simulink model "Framework"  (R2017b)
settings: Solver=ode1  StartTime=0.0  StopTime=Inf  FixedStep=0.001  RelTol=1e-3
PostLoadFcn:
  | , if any(exist('dsrtsu_mdlpostloadfcn', 'file') == [2, 3, 6]), try dsrtsu_mdlpostloadfcn('Execute', bdroot); catch fprintf('Error in PostLoadFcn (dsrtsu_mdlpostloadfcn) for model "%s":\n %s\n', bdroot, lasterr); end, end,
InitFcn:
  | Parameter_INIT
undefined symbols (not defined in the file or in its folder): drive, motor
libraries: rtican x46, simulink x8, neural x1
(part 9 of 10)

== system Framework/rpm FL ==
  Front_Motor_Enable : Inport
  Motor_Output_FL : Inport  Port=2
  Gain1 : Gain
  Terminator_2 : Terminator
  Terminator_3 : Terminator
  Terminator_4 : Terminator
  Transmit OK Detection1 : Subsystem
  _CAN_TYPE1_TX_M1_C2 : rtican/RTICAN Transmit (TX)   Reserved1=[]  Reserved2=[]  Reserved3=[]  Reserved4=[]  SfcnMessage=[]  Msg_Struct=[]  BoardTypeNo=[]  BoardNo=[]  ChannelNo=[]  Parameters=[]  DialogFcn=[]  UnitName=[]  Revision=[]  UnitValues=[]  DSProperties=struct('RTI',struct('Version',uint32(5),'BlockType',struct('isSLSource',uint8(1),'isSLSink',uint8(1),'isHWSource',uint8(0),'isHWSink',uint8(0),'isSetup',uint8(0),'isInline',uint8(1),'isNonInline',uint8(0),'isInterrupt',uint8(0),'isChannelwise',uint8(0)),'IOBoardType','RTICAN','UnitType','MESSAGE','Identifier','TX','DialogType','MSVC','BlockSet','RTICAN','SlaveProcessor','CAN'))  RTIBlockInterface=struct('InputPortsWidth',int32(1),'InputPortsActive',1,'InputPortsName',{{'RPM'}},'InputPortsDataType',{{'SS_DOUBLE'}},'OutputPortsWidth',int32([1 1 1 1]),'OutputPortsActive',[1 1 1 1],'OutputPortsName',{{['TX status'],['TX time'],['TX delta time'],['TX delay time']}},'DialogFcn','rtican_message_interface_gui','BlockDisplay',{{'','center'}},'IconTransparency','on','InitLevel',3,'BlockName',struct('Token',{{'CAN_TYPE','_TX_M','_C'}},'BlockParam',{{'BoardTypeNo','BoardNo','ChannelNo'}}),'SampleTime',{{-1}},'TriggerPort',{{'none'}},'EnablePort',{{'yes'}})  RTIBlockParameters=struct('BoardTypeNo',{{1,'OFF',[]}},'BoardNo',{{1,'ON',[1 16]}},'ChannelNo',{{2,'ON',[1 2]}},'Parameters',{{struct('DataFileSupport',struct('DataFileSelectedMaster',0,'DataFileSelectedLocal',0,'DataFileName',['<no datafile support>|'],'DataFileDate','','SelectedFile',['<no file selected>']),'Options',struct('StatusSelected',1,'TimeSelected',1,'DeltaTimeSelected',1,'DelayTimeSelected',1,'DelayTimeTXCommandSelected',0,'EncodeSetUnusedBitsToOne',0,'EnableMsgLoopback',0,'TriggerPort',struct('Selected',0,'TriggerType',0),'EnablePortSelected',1,'SignalOnPortnameSelected',1,'UserCoding',struct('Selected',0,'InterfaceFile','UserEncodingFile','FcnName','UserEncodeFcn','InportSelected',0,'InportWidth',1,'OutportSelected',0,'OutportWidth',1),'TerminationMsg',struct('Selected',0,'Byte0_7','0'),'InitialMsg',struct('Selected',0,'Byte0_7','0')),'Message',struct('MsgOnBlocknameSelected',0,'MsgName',['TX Message'],'MsgIdFormat',1,'MsgId',780,'MsgLength',4,'NumSignals',1,'SampleTime',-1,'StartTime',struct('Selected',0,'Value',2),'AutoRepeatTime',struct('Selected',0,'Value',0.1),'Timeout',struct('Selected',0,'Value',0.1),'DelayTime',struct('Selected',0,'Value',0.1),'Signal',struct('SgnName','RPM','SgnStartBit',0,'SgnLength',32,'SgnType',0,'ModeValue',-1,'DataType',1,'ByteLayout',1,'Factor',1,'Offset',0,'SgnComment',{{''}},'SgnUnit','','Min',0,'Max',255,'SLDataType','SS_DOUBLE'),'MsgIdNumFormat',1,'MsgComment',{{''}}),'Version',1.2,'general',struct('isFromLib',0)),'OFF',[]}},'GroupId',{{struct('Group',{{'RTICAN'}},'No',2,'Behavior',{{'NAMECHANGE'}},'BlockType',{{'SINK'}},'NameChangeFlag',0),'OFF',[]}},'SFcnRTICANMessage',{{struct('MsgType','TX','SFcnPortType','Scalar','MsgName',['TX Message'],'MsgIdFormat','XTD','MsgId',780,'MsgLength',4,'NumSignals',1,'SampleTime',-1,'StartTime',struct('Selected','no','Value',2),'AutoRepeatTime',struct('Selected','no','Value',0.1),'Timeout',struct('Selected','no','Value',0.1),'Signal',struct('SgnName','RPM','SgnStartBit',0,'SgnLength',32,'SgnType','standard','ModeValue',-1,'DataType',['signed int'],'ByteLayout',['big endian'],'Factor',1,'Offset',0,'SLDataType','SS_DOUBLE'),'StatusSelected','yes','TimeSelected','yes','DeltaTimeSelected','yes','DelayTimeSelected','yes','DelayTimeTXCommandSelected','no','EncodeSetUnusedBitsToOne','no','EnableMsgLoopback','no','TriggerPort',struct('Selected','no','TriggerType',0),'EnablePortSelected','yes','UserCoding',struct('Selected','no','InterfaceFile','UserEncodingFile','FcnName','UserEncodeFcn','InportSelected','no','InportWidth',1,'OutportSelected','no','OutportWidth',1),'TerminationMsg',struct('Selected','no','Byte0','0x00','Byte1','0x00','Byte2','0x00','Byte3','0x00','Byte4','0x00','Byte5','0x00','Byte6','0x00','Byte7','0x00'),'InitialMsg',struct('Selected','no','Byte0','0x00','Byte1','0x00','Byte2','0x00','Byte3','0x00','Byte4','0x00','Byte5','0x00','Byte6','0x00','Byte7','0x00'),'BoardType','DS1','BoardNo',1,'ControllerNo',2),'OFF',[]}},'TLCFileName',{{'rtican_tx_message','OFF',[]}})  RTISFcnParameters=struct('SFcnRTICANMessage','struct','TLCFileName','char')  RTIBlockParaDefault=struct('BoardTypeNo',4302,'BoardNo',1,'ChannelNo',1,'Parameters',struct('DataFileSupport',struct('DataFileSelectedMaster',0,'DataFileSelectedLocal',0,'DataFileName','','DataFileDate','','SelectedFile',['<no file selected>']),'Options',struct('StatusSelected',1,'TimeSelected',1,'DeltaTimeSelected',1,'DelayTimeSelected',1,'DelayTimeTXCommandSelected',0,'EncodeSetUnusedBitsToOne',0,'EnableMsgLoopback',0,'TriggerPort',struct('Selected',0,'TriggerType','rising'),'EnablePortSelected',0,'SignalOnPortnameSelected',1,'UserCoding',struct('Selected',0,'InterfaceFile','UserEncodingFile','FcnName','UserEncodeFcn','InportSelected',0,'InportWidth',1,'OutportSelected',0,'OutportWidth',1),'TerminationMsg',struct('Selected',0,'Byte0_7','0'),'InitialMsg',struct('Selected',0,'Byte0_7','0')),'Message',struct('MsgOnBlocknameSelected',0,'MsgName',['TX Message'],'MsgIdFormat',0,'MsgId',100,'MsgLength',8,'NumSignals',1,'SampleTime',-1,'StartTime',struct('Selected',0,'Value',0),'AutoRepeatTime',struct('Selected',0,'Value',0.1),'Timeout',struct('Selected',0,'Value',0.1),'DelayTime',struct('Selected',0,'Value',0.1),'Signal',struct('SgnName',['TX signal'],'SgnStartBit',0,'SgnLength',8,'SgnType',0,'ModeValue',-1,'DataType',0,'SLDataType','SS_DOUBLE','ByteLayout',0,'Factor',1,'Offset',0,'Min',0,'Max',255,'SgnComment',{{}},'SgnUnit',''),'MsgIdNumFormat',0,'MsgComment',{{''}}),'Version',1.2,'general',struct('isFromLib',1)),'GroupId',struct('Group',{{'RTICAN'}},'No',1,'Behavior',{{'NAMECHANGE'}},'BlockType',{{'SINK'}},'NameChangeFlag',0),'SFcnRTICANMessage',struct('MsgType','TX','MsgName',['TX Message'],'MsgIdFormat','STD','MsgId',100,'MsgLength',2,'NumSignals',1,'SampleTime',-1,'StartTime',struct('Selected','no','Value',0),'AutoRepeatTime',struct('Selected','no','Value',0.1),'Timeout',struct('Selected','no','Value',0.1),'DelayTime',struct('Selected','no','Value',0.1),'Signal',struct('SgnName',['TX signal'],'SgnStartBit',0,'SgnLength',8,'SgnType','standard','ModeValue',-1,'DataType',['unsigned int'],'ByteLayout',['little endian'],'SLDataType','SS_DOUBLE','Factor',1,'Offset',0),'StatusSelected','yes','TimeSelected','yes','DeltaTimeSelected','yes','DelayTimeSelected','yes','EnablePortSelected','no','EnableMsgLoopback','no','DelayTimeTXCommandSelected','no','EncodeSetUnusedBitsToOne','no','UserCoding',struct('Selected','no','InterfaceFile','UserDecodingFile','FcnName','UserDecodeFcn','InportSelected','no','InportWidth',1,'OutportSelected','no','OutportWidth',1),'TerminationMsg',struct('Selected','no','Byte0','0x00','Byte1','0x00','Byte2','0x00','Byte3','0x00','Byte4','0x00','Byte5','0x00','Byte6','0x00','Byte7','0x00'),'InitialMsg',struct('Selected','no','Byte0','0x00','Byte1','0x00','Byte2','0x00','Byte3','0x00','Byte4','0x00','Byte5','0x00','Byte6','0x00','Byte7','0x00'),'TriggerPort',struct('Selected','no','TriggerType','rising'),'BoardType','DS4302','BoardNo',1,'ControllerNo',1,'SFcnPortType','Scalar'),'TLCFileName','rtican_tx_message')
      settings: AttributesFormatString=Group Id: RTICAN2\n  SourceProductName=dSPACE RTI CAN Blockset
  wires:
  Front_Motor_Enable/1 -> _CAN_TYPE1_TX_M1_C2/Enable  "Front_Motor_Enable"
  Motor_Output_FL/1 -> Gain1/1  "Motor_Output_FR"
  _CAN_TYPE1_TX_M1_C2/4 -> Terminator_3/1
  _CAN_TYPE1_TX_M1_C2/3 -> Transmit OK Detection1/2(TX delta time)
  _CAN_TYPE1_TX_M1_C2/1 -> Transmit OK Detection1/1(TX status)
  _CAN_TYPE1_TX_M1_C2/2 -> Terminator_2/1
  Transmit OK Detection1/1(TX Warn) -> Terminator_4/1
  Gain1/1 -> _CAN_TYPE1_TX_M1_C2/1

== system Framework/rpm FR ==
  Front_Motor_Enable : Inport
  Motor_Output_FR : Inport  Port=2
  Gain1 : Gain
  Terminator_2 : Terminator
  Terminator_3 : Terminator
  Terminator_4 : Terminator
  Transmit OK Detection1 : Subsystem
  _CAN_TYPE1_TX_M1_C2 : rtican/RTICAN Transmit (TX)   Reserved1=[]  Reserved2=[]  Reserved3=[]  Reserved4=[]  SfcnMessage=[]  Msg_Struct=[]  BoardTypeNo=[]  BoardNo=[]  ChannelNo=[]  Parameters=[]  DialogFcn=[]  UnitName=[]  Revision=[]  UnitValues=[]  DSProperties=struct('RTI',struct('Version',uint32(5),'BlockType',struct('isSLSource',uint8(1),'isSLSink',uint8(1),'isHWSource',uint8(0),'isHWSink',uint8(0),'isSetup',uint8(0),'isInline',uint8(1),'isNonInline',uint8(0),'isInterrupt',uint8(0),'isChannelwise',uint8(0)),'IOBoardType','RTICAN','UnitType','MESSAGE','Identifier','TX','DialogType','MSVC','BlockSet','RTICAN','SlaveProcessor','CAN'))  RTIBlockInterface=struct('InputPortsWidth',int32(1),'InputPortsActive',1,'InputPortsName',{{'RPM'}},'InputPortsDataType',{{'SS_DOUBLE'}},'OutputPortsWidth',int32([1 1 1 1]),'OutputPortsActive',[1 1 1 1],'OutputPortsName',{{['TX status'],['TX time'],['TX delta time'],['TX delay time']}},'DialogFcn','rtican_message_interface_gui','BlockDisplay',{{'','center'}},'IconTransparency','on','InitLevel',3,'BlockName',struct('Token',{{'CAN_TYPE','_TX_M','_C'}},'BlockParam',{{'BoardTypeNo','BoardNo','ChannelNo'}}),'SampleTime',{{-1}},'TriggerPort',{{'none'}},'EnablePort',{{'yes'}})  RTIBlockParameters=struct('BoardTypeNo',{{1,'OFF',[]}},'BoardNo',{{1,'ON',[1 16]}},'ChannelNo',{{2,'ON',[1 2]}},'Parameters',{{struct('DataFileSupport',struct('DataFileSelectedMaster',0,'DataFileSelectedLocal',0,'DataFileName',['<no datafile support>|'],'DataFileDate','','SelectedFile',['<no file selected>']),'Options',struct('StatusSelected',1,'TimeSelected',1,'DeltaTimeSelected',1,'DelayTimeSelected',1,'DelayTimeTXCommandSelected',0,'EncodeSetUnusedBitsToOne',0,'EnableMsgLoopback',0,'TriggerPort',struct('Selected',0,'TriggerType',0),'EnablePortSelected',1,'SignalOnPortnameSelected',1,'UserCoding',struct('Selected',0,'InterfaceFile','UserEncodingFile','FcnName','UserEncodeFcn','InportSelected',0,'InportWidth',1,'OutportSelected',0,'OutportWidth',1),'TerminationMsg',struct('Selected',0,'Byte0_7','0'),'InitialMsg',struct('Selected',0,'Byte0_7','0')),'Message',struct('MsgOnBlocknameSelected',0,'MsgName',['TX Message'],'MsgIdFormat',1,'MsgId',795,'MsgLength',4,'NumSignals',1,'SampleTime',-1,'StartTime',struct('Selected',0,'Value',2),'AutoRepeatTime',struct('Selected',0,'Value',0.1),'Timeout',struct('Selected',0,'Value',0.1),'DelayTime',struct('Selected',0,'Value',0.1),'Signal',struct('SgnName','RPM','SgnStartBit',0,'SgnLength',32,'SgnType',0,'ModeValue',-1,'DataType',1,'ByteLayout',1,'Factor',1,'Offset',0,'SgnComment',{{''}},'SgnUnit','','Min',0,'Max',255,'SLDataType','SS_DOUBLE'),'MsgIdNumFormat',1,'MsgComment',{{''}}),'Version',1.2,'general',struct('isFromLib',0)),'OFF',[]}},'GroupId',{{struct('Group',{{'RTICAN'}},'No',2,'Behavior',{{'NAMECHANGE'}},'BlockType',{{'SINK'}},'NameChangeFlag',0),'OFF',[]}},'SFcnRTICANMessage',{{struct('MsgType','TX','SFcnPortType','Scalar','MsgName',['TX Message'],'MsgIdFormat','XTD','MsgId',795,'MsgLength',4,'NumSignals',1,'SampleTime',-1,'StartTime',struct('Selected','no','Value',2),'AutoRepeatTime',struct('Selected','no','Value',0.1),'Timeout',struct('Selected','no','Value',0.1),'Signal',struct('SgnName','RPM','SgnStartBit',0,'SgnLength',32,'SgnType','standard','ModeValue',-1,'DataType',['signed int'],'ByteLayout',['big endian'],'Factor',1,'Offset',0,'SLDataType','SS_DOUBLE'),'StatusSelected','yes','TimeSelected','yes','DeltaTimeSelected','yes','DelayTimeSelected','yes','DelayTimeTXCommandSelected','no','EncodeSetUnusedBitsToOne','no','EnableMsgLoopback','no','TriggerPort',struct('Selected','no','TriggerType',0),'EnablePortSelected','yes','UserCoding',struct('Selected','no','InterfaceFile','UserEncodingFile','FcnName','UserEncodeFcn','InportSelected','no','InportWidth',1,'OutportSelected','no','OutportWidth',1),'TerminationMsg',struct('Selected','no','Byte0','0x00','Byte1','0x00','Byte2','0x00','Byte3','0x00','Byte4','0x00','Byte5','0x00','Byte6','0x00','Byte7','0x00'),'InitialMsg',struct('Selected','no','Byte0','0x00','Byte1','0x00','Byte2','0x00','Byte3','0x00','Byte4','0x00','Byte5','0x00','Byte6','0x00','Byte7','0x00'),'BoardType','DS1','BoardNo',1,'ControllerNo',2),'OFF',[]}},'TLCFileName',{{'rtican_tx_message','OFF',[]}})  RTISFcnParameters=struct('SFcnRTICANMessage','struct','TLCFileName','char')  RTIBlockParaDefault=struct('BoardTypeNo',4302,'BoardNo',1,'ChannelNo',1,'Parameters',struct('DataFileSupport',struct('DataFileSelectedMaster',0,'DataFileSelectedLocal',0,'DataFileName','','DataFileDate','','SelectedFile',['<no file selected>']),'Options',struct('StatusSelected',1,'TimeSelected',1,'DeltaTimeSelected',1,'DelayTimeSelected',1,'DelayTimeTXCommandSelected',0,'EncodeSetUnusedBitsToOne',0,'EnableMsgLoopback',0,'TriggerPort',struct('Selected',0,'TriggerType','rising'),'EnablePortSelected',0,'SignalOnPortnameSelected',1,'UserCoding',struct('Selected',0,'InterfaceFile','UserEncodingFile','FcnName','UserEncodeFcn','InportSelected',0,'InportWidth',1,'OutportSelected',0,'OutportWidth',1),'TerminationMsg',struct('Selected',0,'Byte0_7','0'),'InitialMsg',struct('Selected',0,'Byte0_7','0')),'Message',struct('MsgOnBlocknameSelected',0,'MsgName',['TX Message'],'MsgIdFormat',0,'MsgId',100,'MsgLength',8,'NumSignals',1,'SampleTime',-1,'StartTime',struct('Selected',0,'Value',0),'AutoRepeatTime',struct('Selected',0,'Value',0.1),'Timeout',struct('Selected',0,'Value',0.1),'DelayTime',struct('Selected',0,'Value',0.1),'Signal',struct('SgnName',['TX signal'],'SgnStartBit',0,'SgnLength',8,'SgnType',0,'ModeValue',-1,'DataType',0,'SLDataType','SS_DOUBLE','ByteLayout',0,'Factor',1,'Offset',0,'Min',0,'Max',255,'SgnComment',{{}},'SgnUnit',''),'MsgIdNumFormat',0,'MsgComment',{{''}}),'Version',1.2,'general',struct('isFromLib',1)),'GroupId',struct('Group',{{'RTICAN'}},'No',1,'Behavior',{{'NAMECHANGE'}},'BlockType',{{'SINK'}},'NameChangeFlag',0),'SFcnRTICANMessage',struct('MsgType','TX','MsgName',['TX Message'],'MsgIdFormat','STD','MsgId',100,'MsgLength',2,'NumSignals',1,'SampleTime',-1,'StartTime',struct('Selected','no','Value',0),'AutoRepeatTime',struct('Selected','no','Value',0.1),'Timeout',struct('Selected','no','Value',0.1),'DelayTime',struct('Selected','no','Value',0.1),'Signal',struct('SgnName',['TX signal'],'SgnStartBit',0,'SgnLength',8,'SgnType','standard','ModeValue',-1,'DataType',['unsigned int'],'ByteLayout',['little endian'],'SLDataType','SS_DOUBLE','Factor',1,'Offset',0),'StatusSelected','yes','TimeSelected','yes','DeltaTimeSelected','yes','DelayTimeSelected','yes','EnablePortSelected','no','EnableMsgLoopback','no','DelayTimeTXCommandSelected','no','EncodeSetUnusedBitsToOne','no','UserCoding',struct('Selected','no','InterfaceFile','UserDecodingFile','FcnName','UserDecodeFcn','InportSelected','no','InportWidth',1,'OutportSelected','no','OutportWidth',1),'TerminationMsg',struct('Selected','no','Byte0','0x00','Byte1','0x00','Byte2','0x00','Byte3','0x00','Byte4','0x00','Byte5','0x00','Byte6','0x00','Byte7','0x00'),'InitialMsg',struct('Selected','no','Byte0','0x00','Byte1','0x00','Byte2','0x00','Byte3','0x00','Byte4','0x00','Byte5','0x00','Byte6','0x00','Byte7','0x00'),'TriggerPort',struct('Selected','no','TriggerType','rising'),'BoardType','DS4302','BoardNo',1,'ControllerNo',1,'SFcnPortType','Scalar'),'TLCFileName','rtican_tx_message')
      settings: AttributesFormatString=Group Id: RTICAN2\n  SourceProductName=dSPACE RTI CAN Blockset
  wires:
  Front_Motor_Enable/1 -> _CAN_TYPE1_TX_M1_C2/Enable  "Front_Motor_Enable"
  Motor_Output_FR/1 -> Gain1/1  "Motor_Output_FR"
  _CAN_TYPE1_TX_M1_C2/4 -> Terminator_3/1
  _CAN_TYPE1_TX_M1_C2/3 -> Transmit OK Detection1/2(TX delta time)
  _CAN_TYPE1_TX_M1_C2/1 -> Transmit OK Detection1/1(TX status)
  _CAN_TYPE1_TX_M1_C2/2 -> Terminator_2/1
  Transmit OK Detection1/1(TX Warn) -> Terminator_4/1
  Gain1/1 -> _CAN_TYPE1_TX_M1_C2/1

== system Framework/rpm RL ==
  Front_Motor_Enable : Inport
  Motor_Output_RL : Inport  Port=2
  Gain1 : Gain
  Terminator_2 : Terminator
  Terminator_3 : Terminator
  Terminator_4 : Terminator
  Transmit OK Detection1 : Subsystem
  _CAN_TYPE1_TX_M1_C2 : rtican/RTICAN Transmit (TX)   Reserved1=[]  Reserved2=[]  Reserved3=[]  Reserved4=[]  SfcnMessage=[]  Msg_Struct=[]  BoardTypeNo=[]  BoardNo=[]  ChannelNo=[]  Parameters=[]  DialogFcn=[]  UnitName=[]  Revision=[]  UnitValues=[]  DSProperties=struct('RTI',struct('Version',uint32(5),'BlockType',struct('isSLSource',uint8(1),'isSLSink',uint8(1),'isHWSource',uint8(0),'isHWSink',uint8(0),'isSetup',uint8(0),'isInline',uint8(1),'isNonInline',uint8(0),'isInterrupt',uint8(0),'isChannelwise',uint8(0)),'IOBoardType','RTICAN','UnitType','MESSAGE','Identifier','TX','DialogType','MSVC','BlockSet','RTICAN','SlaveProcessor','CAN'))  RTIBlockInterface=struct('InputPortsWidth',int32(1),'InputPortsActive',1,'InputPortsName',{{'RPM'}},'InputPortsDataType',{{'SS_DOUBLE'}},'OutputPortsWidth',int32([1 1 1 1]),'OutputPortsActive',[1 1 1 1],'OutputPortsName',{{['TX status'],['TX time'],['TX delta time'],['TX delay time']}},'DialogFcn','rtican_message_interface_gui','BlockDisplay',{{'','center'}},'IconTransparency','on','InitLevel',3,'BlockName',struct('Token',{{'CAN_TYPE','_TX_M','_C'}},'BlockParam',{{'BoardTypeNo','BoardNo','ChannelNo'}}),'SampleTime',{{-1}},'TriggerPort',{{'none'}},'EnablePort',{{'yes'}})  RTIBlockParameters=struct('BoardTypeNo',{{1,'OFF',[]}},'BoardNo',{{1,'ON',[1 16]}},'ChannelNo',{{2,'ON',[1 2]}},'Parameters',{{struct('DataFileSupport',struct('DataFileSelectedMaster',0,'DataFileSelectedLocal',0,'DataFileName',['<no datafile support>|'],'DataFileDate','','SelectedFile',['<no file selected>']),'Options',struct('StatusSelected',1,'TimeSelected',1,'DeltaTimeSelected',1,'DelayTimeSelected',1,'DelayTimeTXCommandSelected',0,'EncodeSetUnusedBitsToOne',0,'EnableMsgLoopback',0,'TriggerPort',struct('Selected',0,'TriggerType',0),'EnablePortSelected',1,'SignalOnPortnameSelected',1,'UserCoding',struct('Selected',0,'InterfaceFile','UserEncodingFile','FcnName','UserEncodeFcn','InportSelected',0,'InportWidth',1,'OutportSelected',0,'OutportWidth',1),'TerminationMsg',struct('Selected',0,'Byte0_7','0'),'InitialMsg',struct('Selected',0,'Byte0_7','0')),'Message',struct('MsgOnBlocknameSelected',0,'MsgName',['TX Message'],'MsgIdFormat',1,'MsgId',848,'MsgLength',4,'NumSignals',1,'SampleTime',-1,'StartTime',struct('Selected',0,'Value',2),'AutoRepeatTime',struct('Selected',0,'Value',0.1),'Timeout',struct('Selected',0,'Value',0.1),'DelayTime',struct('Selected',0,'Value',0.1),'Signal',struct('SgnName','RPM','SgnStartBit',0,'SgnLength',32,'SgnType',0,'ModeValue',-1,'DataType',1,'ByteLayout',1,'Factor',1,'Offset',0,'SgnComment',{{''}},'SgnUnit','','Min',0,'Max',255,'SLDataType','SS_DOUBLE'),'MsgIdNumFormat',1,'MsgComment',{{''}}),'Version',1.2,'general',struct('isFromLib',0)),'OFF',[]}},'GroupId',{{struct('Group',{{'RTICAN'}},'No',2,'Behavior',{{'NAMECHANGE'}},'BlockType',{{'SINK'}},'NameChangeFlag',0),'OFF',[]}},'SFcnRTICANMessage',{{struct('MsgType','TX','SFcnPortType','Scalar','MsgName',['TX Message'],'MsgIdFormat','XTD','MsgId',848,'MsgLength',4,'NumSignals',1,'SampleTime',-1,'StartTime',struct('Selected','no','Value',2),'AutoRepeatTime',struct('Selected','no','Value',0.1),'Timeout',struct('Selected','no','Value',0.1),'Signal',struct('SgnName','RPM','SgnStartBit',0,'SgnLength',32,'SgnType','standard','ModeValue',-1,'DataType',['signed int'],'ByteLayout',['big endian'],'Factor',1,'Offset',0,'SLDataType','SS_DOUBLE'),'StatusSelected','yes','TimeSelected','yes','DeltaTimeSelected','yes','DelayTimeSelected','yes','DelayTimeTXCommandSelected','no','EncodeSetUnusedBitsToOne','no','EnableMsgLoopback','no','TriggerPort',struct('Selected','no','TriggerType',0),'EnablePortSelected','yes','UserCoding',struct('Selected','no','InterfaceFile','UserEncodingFile','FcnName','UserEncodeFcn','InportSelected','no','InportWidth',1,'OutportSelected','no','OutportWidth',1),'TerminationMsg',struct('Selected','no','Byte0','0x00','Byte1','0x00','Byte2','0x00','Byte3','0x00','Byte4','0x00','Byte5','0x00','Byte6','0x00','Byte7','0x00'),'InitialMsg',struct('Selected','no','Byte0','0x00','Byte1','0x00','Byte2','0x00','Byte3','0x00','Byte4','0x00','Byte5','0x00','Byte6','0x00','Byte7','0x00'),'BoardType','DS1','BoardNo',1,'ControllerNo',2),'OFF',[]}},'TLCFileName',{{'rtican_tx_message','OFF',[]}})  RTISFcnParameters=struct('SFcnRTICANMessage','struct','TLCFileName','char')  RTIBlockParaDefault=struct('BoardTypeNo',4302,'BoardNo',1,'ChannelNo',1,'Parameters',struct('DataFileSupport',struct('DataFileSelectedMaster',0,'DataFileSelectedLocal',0,'DataFileName','','DataFileDate','','SelectedFile',['<no file selected>']),'Options',struct('StatusSelected',1,'TimeSelected',1,'DeltaTimeSelected',1,'DelayTimeSelected',1,'DelayTimeTXCommandSelected',0,'EncodeSetUnusedBitsToOne',0,'EnableMsgLoopback',0,'TriggerPort',struct('Selected',0,'TriggerType','rising'),'EnablePortSelected',0,'SignalOnPortnameSelected',1,'UserCoding',struct('Selected',0,'InterfaceFile','UserEncodingFile','FcnName','UserEncodeFcn','InportSelected',0,'InportWidth',1,'OutportSelected',0,'OutportWidth',1),'TerminationMsg',struct('Selected',0,'Byte0_7','0'),'InitialMsg',struct('Selected',0,'Byte0_7','0')),'Message',struct('MsgOnBlocknameSelected',0,'MsgName',['TX Message'],'MsgIdFormat',0,'MsgId',100,'MsgLength',8,'NumSignals',1,'SampleTime',-1,'StartTime',struct('Selected',0,'Value',0),'AutoRepeatTime',struct('Selected',0,'Value',0.1),'Timeout',struct('Selected',0,'Value',0.1),'DelayTime',struct('Selected',0,'Value',0.1),'Signal',struct('SgnName',['TX signal'],'SgnStartBit',0,'SgnLength',8,'SgnType',0,'ModeValue',-1,'DataType',0,'SLDataType','SS_DOUBLE','ByteLayout',0,'Factor',1,'Offset',0,'Min',0,'Max',255,'SgnComment',{{}},'SgnUnit',''),'MsgIdNumFormat',0,'MsgComment',{{''}}),'Version',1.2,'general',struct('isFromLib',1)),'GroupId',struct('Group',{{'RTICAN'}},'No',1,'Behavior',{{'NAMECHANGE'}},'BlockType',{{'SINK'}},'NameChangeFlag',0),'SFcnRTICANMessage',struct('MsgType','TX','MsgName',['TX Message'],'MsgIdFormat','STD','MsgId',100,'MsgLength',2,'NumSignals',1,'SampleTime',-1,'StartTime',struct('Selected','no','Value',0),'AutoRepeatTime',struct('Selected','no','Value',0.1),'Timeout',struct('Selected','no','Value',0.1),'DelayTime',struct('Selected','no','Value',0.1),'Signal',struct('SgnName',['TX signal'],'SgnStartBit',0,'SgnLength',8,'SgnType','standard','ModeValue',-1,'DataType',['unsigned int'],'ByteLayout',['little endian'],'SLDataType','SS_DOUBLE','Factor',1,'Offset',0),'StatusSelected','yes','TimeSelected','yes','DeltaTimeSelected','yes','DelayTimeSelected','yes','EnablePortSelected','no','EnableMsgLoopback','no','DelayTimeTXCommandSelected','no','EncodeSetUnusedBitsToOne','no','UserCoding',struct('Selected','no','InterfaceFile','UserDecodingFile','FcnName','UserDecodeFcn','InportSelected','no','InportWidth',1,'OutportSelected','no','OutportWidth',1),'TerminationMsg',struct('Selected','no','Byte0','0x00','Byte1','0x00','Byte2','0x00','Byte3','0x00','Byte4','0x00','Byte5','0x00','Byte6','0x00','Byte7','0x00'),'InitialMsg',struct('Selected','no','Byte0','0x00','Byte1','0x00','Byte2','0x00','Byte3','0x00','Byte4','0x00','Byte5','0x00','Byte6','0x00','Byte7','0x00'),'TriggerPort',struct('Selected','no','TriggerType','rising'),'BoardType','DS4302','BoardNo',1,'ControllerNo',1,'SFcnPortType','Scalar'),'TLCFileName','rtican_tx_message')
      settings: AttributesFormatString=Group Id: RTICAN2\n  SourceProductName=dSPACE RTI CAN Blockset
  wires:
  Front_Motor_Enable/1 -> _CAN_TYPE1_TX_M1_C2/Enable  "Front_Motor_Enable"
  Motor_Output_RL/1 -> Gain1/1  "Motor_Output_FR"
  _CAN_TYPE1_TX_M1_C2/4 -> Terminator_3/1
  _CAN_TYPE1_TX_M1_C2/3 -> Transmit OK Detection1/2(TX delta time)
  _CAN_TYPE1_TX_M1_C2/1 -> Transmit OK Detection1/1(TX status)
  _CAN_TYPE1_TX_M1_C2/2 -> Terminator_2/1
  Transmit OK Detection1/1(TX Warn) -> Terminator_4/1
  Gain1/1 -> _CAN_TYPE1_TX_M1_C2/1

== system Framework/rpm RR ==
  Front_Motor_Enable : Inport
  Motor_Output_RR : Inport  Port=2
  Gain1 : Gain
  Terminator_2 : Terminator
  Terminator_3 : Terminator
  Terminator_4 : Terminator
  Transmit OK Detection1 : Subsystem
  _CAN_TYPE1_TX_M1_C2 : rtican/RTICAN Transmit (TX)   Reserved1=[]  Reserved2=[]  Reserved3=[]  Reserved4=[]  SfcnMessage=[]  Msg_Struct=[]  BoardTypeNo=[]  BoardNo=[]  ChannelNo=[]  Parameters=[]  DialogFcn=[]  UnitName=[]  Revision=[]  UnitValues=[]  DSProperties=struct('RTI',struct('Version',uint32(5),'BlockType',struct('isSLSource',uint8(1),'isSLSink',uint8(1),'isHWSource',uint8(0),'isHWSink',uint8(0),'isSetup',uint8(0),'isInline',uint8(1),'isNonInline',uint8(0),'isInterrupt',uint8(0),'isChannelwise',uint8(0)),'IOBoardType','RTICAN','UnitType','MESSAGE','Identifier','TX','DialogType','MSVC','BlockSet','RTICAN','SlaveProcessor','CAN'))  RTIBlockInterface=struct('InputPortsWidth',int32(1),'InputPortsActive',1,'InputPortsName',{{'RPM'}},'InputPortsDataType',{{'SS_DOUBLE'}},'OutputPortsWidth',int32([1 1 1 1]),'OutputPortsActive',[1 1 1 1],'OutputPortsName',{{['TX status'],['TX time'],['TX delta time'],['TX delay time']}},'DialogFcn','rtican_message_interface_gui','BlockDisplay',{{'','center'}},'IconTransparency','on','InitLevel',3,'BlockName',struct('Token',{{'CAN_TYPE','_TX_M','_C'}},'BlockParam',{{'BoardTypeNo','BoardNo','ChannelNo'}}),'SampleTime',{{-1}},'TriggerPort',{{'none'}},'EnablePort',{{'yes'}})  RTIBlockParameters=struct('BoardTypeNo',{{1,'OFF',[]}},'BoardNo',{{1,'ON',[1 16]}},'ChannelNo',{{2,'ON',[1 2]}},'Parameters',{{struct('DataFileSupport',struct('DataFileSelectedMaster',0,'DataFileSelectedLocal',0,'DataFileName',['<no datafile support>|'],'DataFileDate','','SelectedFile',['<no file selected>']),'Options',struct('StatusSelected',1,'TimeSelected',1,'DeltaTimeSelected',1,'DelayTimeSelected',1,'DelayTimeTXCommandSelected',0,'EncodeSetUnusedBitsToOne',0,'EnableMsgLoopback',0,'TriggerPort',struct('Selected',0,'TriggerType',0),'EnablePortSelected',1,'SignalOnPortnameSelected',1,'UserCoding',struct('Selected',0,'InterfaceFile','UserEncodingFile','FcnName','UserEncodeFcn','InportSelected',0,'InportWidth',1,'OutportSelected',0,'OutportWidth',1),'TerminationMsg',struct('Selected',0,'Byte0_7','0'),'InitialMsg',struct('Selected',0,'Byte0_7','0')),'Message',struct('MsgOnBlocknameSelected',0,'MsgName',['TX Message'],'MsgIdFormat',1,'MsgId',851,'MsgLength',4,'NumSignals',1,'SampleTime',-1,'StartTime',struct('Selected',0,'Value',2),'AutoRepeatTime',struct('Selected',0,'Value',0.1),'Timeout',struct('Selected',0,'Value',0.1),'DelayTime',struct('Selected',0,'Value',0.1),'Signal',struct('SgnName','RPM','SgnStartBit',0,'SgnLength',32,'SgnType',0,'ModeValue',-1,'DataType',1,'ByteLayout',1,'Factor',1,'Offset',0,'SgnComment',{{''}},'SgnUnit','','Min',0,'Max',255,'SLDataType','SS_DOUBLE'),'MsgIdNumFormat',1,'MsgComment',{{''}}),'Version',1.2,'general',struct('isFromLib',0)),'OFF',[]}},'GroupId',{{struct('Group',{{'RTICAN'}},'No',2,'Behavior',{{'NAMECHANGE'}},'BlockType',{{'SINK'}},'NameChangeFlag',0),'OFF',[]}},'SFcnRTICANMessage',{{struct('MsgType','TX','SFcnPortType','Scalar','MsgName',['TX Message'],'MsgIdFormat','XTD','MsgId',851,'MsgLength',4,'NumSignals',1,'SampleTime',-1,'StartTime',struct('Selected','no','Value',2),'AutoRepeatTime',struct('Selected','no','Value',0.1),'Timeout',struct('Selected','no','Value',0.1),'Signal',struct('SgnName','RPM','SgnStartBit',0,'SgnLength',32,'SgnType','standard','ModeValue',-1,'DataType',['signed int'],'ByteLayout',['big endian'],'Factor',1,'Offset',0,'SLDataType','SS_DOUBLE'),'StatusSelected','yes','TimeSelected','yes','DeltaTimeSelected','yes','DelayTimeSelected','yes','DelayTimeTXCommandSelected','no','EncodeSetUnusedBitsToOne','no','EnableMsgLoopback','no','TriggerPort',struct('Selected','no','TriggerType',0),'EnablePortSelected','yes','UserCoding',struct('Selected','no','InterfaceFile','UserEncodingFile','FcnName','UserEncodeFcn','InportSelected','no','InportWidth',1,'OutportSelected','no','OutportWidth',1),'TerminationMsg',struct('Selected','no','Byte0','0x00','Byte1','0x00','Byte2','0x00','Byte3','0x00','Byte4','0x00','Byte5','0x00','Byte6','0x00','Byte7','0x00'),'InitialMsg',struct('Selected','no','Byte0','0x00','Byte1','0x00','Byte2','0x00','Byte3','0x00','Byte4','0x00','Byte5','0x00','Byte6','0x00','Byte7','0x00'),'BoardType','DS1','BoardNo',1,'ControllerNo',2),'OFF',[]}},'TLCFileName',{{'rtican_tx_message','OFF',[]}})  RTISFcnParameters=struct('SFcnRTICANMessage','struct','TLCFileName','char')  RTIBlockParaDefault=struct('BoardTypeNo',4302,'BoardNo',1,'ChannelNo',1,'Parameters',struct('DataFileSupport',struct('DataFileSelectedMaster',0,'DataFileSelectedLocal',0,'DataFileName','','DataFileDate','','SelectedFile',['<no file selected>']),'Options',struct('StatusSelected',1,'TimeSelected',1,'DeltaTimeSelected',1,'DelayTimeSelected',1,'DelayTimeTXCommandSelected',0,'EncodeSetUnusedBitsToOne',0,'EnableMsgLoopback',0,'TriggerPort',struct('Selected',0,'TriggerType','rising'),'EnablePortSelected',0,'SignalOnPortnameSelected',1,'UserCoding',struct('Selected',0,'InterfaceFile','UserEncodingFile','FcnName','UserEncodeFcn','InportSelected',0,'InportWidth',1,'OutportSelected',0,'OutportWidth',1),'TerminationMsg',struct('Selected',0,'Byte0_7','0'),'InitialMsg',struct('Selected',0,'Byte0_7','0')),'Message',struct('MsgOnBlocknameSelected',0,'MsgName',['TX Message'],'MsgIdFormat',0,'MsgId',100,'MsgLength',8,'NumSignals',1,'SampleTime',-1,'StartTime',struct('Selected',0,'Value',0),'AutoRepeatTime',struct('Selected',0,'Value',0.1),'Timeout',struct('Selected',0,'Value',0.1),'DelayTime',struct('Selected',0,'Value',0.1),'Signal',struct('SgnName',['TX signal'],'SgnStartBit',0,'SgnLength',8,'SgnType',0,'ModeValue',-1,'DataType',0,'SLDataType','SS_DOUBLE','ByteLayout',0,'Factor',1,'Offset',0,'Min',0,'Max',255,'SgnComment',{{}},'SgnUnit',''),'MsgIdNumFormat',0,'MsgComment',{{''}}),'Version',1.2,'general',struct('isFromLib',1)),'GroupId',struct('Group',{{'RTICAN'}},'No',1,'Behavior',{{'NAMECHANGE'}},'BlockType',{{'SINK'}},'NameChangeFlag',0),'SFcnRTICANMessage',struct('MsgType','TX','MsgName',['TX Message'],'MsgIdFormat','STD','MsgId',100,'MsgLength',2,'NumSignals',1,'SampleTime',-1,'StartTime',struct('Selected','no','Value',0),'AutoRepeatTime',struct('Selected','no','Value',0.1),'Timeout',struct('Selected','no','Value',0.1),'DelayTime',struct('Selected','no','Value',0.1),'Signal',struct('SgnName',['TX signal'],'SgnStartBit',0,'SgnLength',8,'SgnType','standard','ModeValue',-1,'DataType',['unsigned int'],'ByteLayout',['little endian'],'SLDataType','SS_DOUBLE','Factor',1,'Offset',0),'StatusSelected','yes','TimeSelected','yes','DeltaTimeSelected','yes','DelayTimeSelected','yes','EnablePortSelected','no','EnableMsgLoopback','no','DelayTimeTXCommandSelected','no','EncodeSetUnusedBitsToOne','no','UserCoding',struct('Selected','no','InterfaceFile','UserDecodingFile','FcnName','UserDecodeFcn','InportSelected','no','InportWidth',1,'OutportSelected','no','OutportWidth',1),'TerminationMsg',struct('Selected','no','Byte0','0x00','Byte1','0x00','Byte2','0x00','Byte3','0x00','Byte4','0x00','Byte5','0x00','Byte6','0x00','Byte7','0x00'),'InitialMsg',struct('Selected','no','Byte0','0x00','Byte1','0x00','Byte2','0x00','Byte3','0x00','Byte4','0x00','Byte5','0x00','Byte6','0x00','Byte7','0x00'),'TriggerPort',struct('Selected','no','TriggerType','rising'),'BoardType','DS4302','BoardNo',1,'ControllerNo',1,'SFcnPortType','Scalar'),'TLCFileName','rtican_tx_message')
      settings: AttributesFormatString=Group Id: RTICAN2\n  SourceProductName=dSPACE RTI CAN Blockset
  wires:
  Front_Motor_Enable/1 -> _CAN_TYPE1_TX_M1_C2/Enable  "Front_Motor_Enable"
  Motor_Output_RR/1 -> Gain1/1  "Motor_Output_FR"
  _CAN_TYPE1_TX_M1_C2/4 -> Terminator_3/1
  _CAN_TYPE1_TX_M1_C2/3 -> Transmit OK Detection1/2(TX delta time)
  _CAN_TYPE1_TX_M1_C2/1 -> Transmit OK Detection1/1(TX status)
  _CAN_TYPE1_TX_M1_C2/2 -> Terminator_2/1
  Transmit OK Detection1/1(TX Warn) -> Terminator_4/1
  Gain1/1 -> _CAN_TYPE1_TX_M1_C2/1

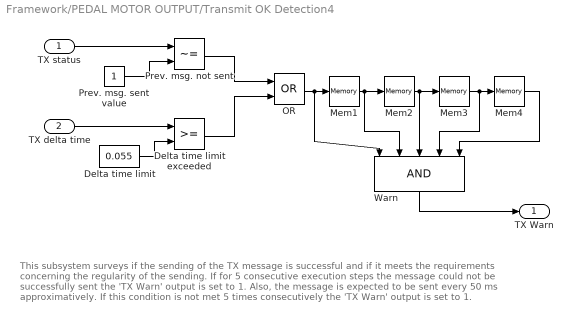
== system Framework/PEDAL MOTOR OUTPUT/Transmit OK Detection4 ==
  note: This subsystem surveys if the sending of the TX message is successful and if it meets the
      | requirements concerning the regularity of the sending.
      |
      | If for 5 consecutive execution steps the message could not be successfully sent the 'TX Warn'
      | output is set to 1. Also, the message is expected to be sent every 50 ms approximatively. If this
      | condition is not met 5 times consecutively the 'TX Warn' output is set to 1.
  TX status : Inport
  TX delta time : Inport  Port=2
  Delta time limit : Constant  Value=0.055
  Delta time limit exceeded : RelationalOperator  RndMeth=Nearest  InputSameDT=on
  Mem{1..4} (4 alike) : Memory
  OR : Logic  Operator=OR
  Prev. msg. not sent : RelationalOperator  Operator=~=  RndMeth=Nearest  InputSameDT=on
  Prev. msg. sent value : Constant
  Warn : Logic  Inputs=5
  TX Warn : Outport
  wires:
  TX delta time/1 -> Delta time limit exceeded/1
  Delta time limit/1 -> Delta time limit exceeded/2
  Prev. msg. sent value/1 -> Prev. msg. not sent/2
  TX status/1 -> Prev. msg. not sent/1
  Prev. msg. not sent/1 -> OR/1
  Delta time limit exceeded/1 -> OR/2
  OR/1 -> Mem1/1, Warn/1
  Mem1/1 -> Mem2/1, Warn/2
  Mem2/1 -> Mem3/1, Warn/3
  Mem3/1 -> Mem4/1, Warn/4
  Mem4/1 -> Warn/5
  Warn/1 -> TX Warn/1

== system Framework/RTI Data/RTI Data Store ==
  RTI Data Store : Subsystem  mask(RTI_DATA_STORE){}
      mask help:
      | RTI Data Store Block. This block is used by RTI to store internal model dependent data. Deleting this block will result in data loss.
      |
      | NEVER DELETE, COPY, OR MODIFY THIS BLOCK!
      mask Help:
      | RTI Data Store Block. This block is used by RTI to store internal model dependent data. Deleting this block will result in data loss.
      | 
      | NEVER DELETE, COPY, OR MODIFY THIS BLOCK!
      mask Display: text(0.5, 0.5, ' ', 'HorizontalAlignment', 'center');

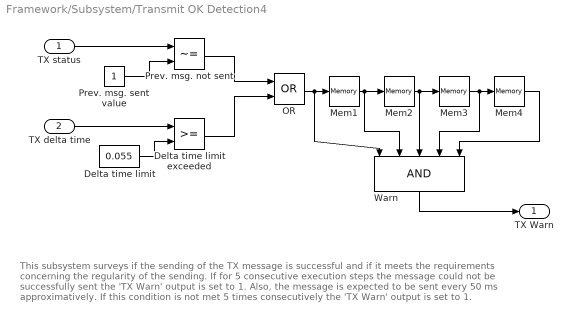
== system Framework/Subsystem/Transmit OK Detection4 ==
  note: This subsystem surveys if the sending of the TX message is successful and if it meets the
      | requirements concerning the regularity of the sending.
      |
      | If for 5 consecutive execution steps the message could not be successfully sent the 'TX Warn'
      | output is set to 1. Also, the message is expected to be sent every 50 ms approximatively. If this
      | condition is not met 5 times consecutively the 'TX Warn' output is set to 1.
  TX status : Inport
  TX delta time : Inport  Port=2
  Delta time limit : Constant  Value=0.055
  Delta time limit exceeded : RelationalOperator  RndMeth=Nearest  InputSameDT=on
  Mem{1..4} (4 alike) : Memory
  OR : Logic  Operator=OR
  Prev. msg. not sent : RelationalOperator  Operator=~=  RndMeth=Nearest  InputSameDT=on
  Prev. msg. sent value : Constant
  Warn : Logic  Inputs=5
  TX Warn : Outport
  wires:
  TX delta time/1 -> Delta time limit exceeded/1
  Delta time limit/1 -> Delta time limit exceeded/2
  Prev. msg. sent value/1 -> Prev. msg. not sent/2
  TX status/1 -> Prev. msg. not sent/1
  Prev. msg. not sent/1 -> OR/1
  Delta time limit exceeded/1 -> OR/2
  OR/1 -> Mem1/1, Warn/1
  Mem1/1 -> Mem2/1, Warn/2
  Mem2/1 -> Mem3/1, Warn/3
  Mem3/1 -> Mem4/1, Warn/4
  Mem4/1 -> Warn/5
  Warn/1 -> TX Warn/1

== system Framework/Subsystem/Transmit OK Detection6 ==
  note: This subsystem surveys if the sending of the TX message is successful and if it meets the
      | requirements concerning the regularity of the sending.
      |
      | If for 5 consecutive execution steps the message could not be successfully sent the 'TX Warn'
      | output is set to 1. Also, the message is expected to be sent every 50 ms approximatively. If this
      | condition is not met 5 times consecutively the 'TX Warn' output is set to 1.
  TX status : Inport
  TX delta time : Inport  Port=2
  Delta time limit : Constant  Value=0.055
  Delta time limit exceeded : RelationalOperator  RndMeth=Nearest  InputSameDT=on
  Mem{1..4} (4 alike) : Memory
  OR : Logic  Operator=OR
  Prev. msg. not sent : RelationalOperator  Operator=~=  RndMeth=Nearest  InputSameDT=on
  Prev. msg. sent value : Constant
  Warn : Logic  Inputs=5
  TX Warn : Outport
  wires:
  TX delta time/1 -> Delta time limit exceeded/1
  Delta time limit/1 -> Delta time limit exceeded/2
  Prev. msg. sent value/1 -> Prev. msg. not sent/2
  TX status/1 -> Prev. msg. not sent/1
  Prev. msg. not sent/1 -> OR/1
  Delta time limit exceeded/1 -> OR/2
  OR/1 -> Mem1/1, Warn/1
  Mem1/1 -> Mem2/1, Warn/2
  Mem2/1 -> Mem3/1, Warn/3
  Mem3/1 -> Mem4/1, Warn/4
  Mem4/1 -> Warn/5
  Warn/1 -> TX Warn/1

== system Framework/Subsystem1/Transmit OK Detection1 ==
  note: This subsystem surveys if the sending of the TX message is successful and if it meets the
      | requirements concerning the regularity of the sending.
      |
      | If for 5 consecutive execution steps the message could not be successfully sent the 'TX Warn'
      | output is set to 1. Also, the message is expected to be sent every 50 ms approximatively. If this
      | condition is not met 5 times consecutively the 'TX Warn' output is set to 1.
  TX status : Inport
  TX delta time : Inport  Port=2
  Delta time limit : Constant  Value=0.055
  Delta time limit exceeded : RelationalOperator  RndMeth=Nearest  InputSameDT=on
  Mem{1..4} (4 alike) : Memory
  OR : Logic  Operator=OR
  Prev. msg. not sent : RelationalOperator  Operator=~=  RndMeth=Nearest  InputSameDT=on
  Prev. msg. sent value : Constant
  Warn : Logic  Inputs=5
  TX Warn : Outport
  wires:
  TX delta time/1 -> Delta time limit exceeded/1
  Delta time limit/1 -> Delta time limit exceeded/2
  Prev. msg. sent value/1 -> Prev. msg. not sent/2
  TX status/1 -> Prev. msg. not sent/1
  Prev. msg. not sent/1 -> OR/1
  Delta time limit exceeded/1 -> OR/2
  OR/1 -> Mem1/1, Warn/1
  Mem1/1 -> Mem2/1, Warn/2
  Mem2/1 -> Mem3/1, Warn/3
  Mem3/1 -> Mem4/1, Warn/4
  Mem4/1 -> Warn/5
  Warn/1 -> TX Warn/1

== system Framework/Subsystem1/Transmit OK Detection5 ==
  note: This subsystem surveys if the sending of the TX message is successful and if it meets the
      | requirements concerning the regularity of the sending.
      |
      | If for 5 consecutive execution steps the message could not be successfully sent the 'TX Warn'
      | output is set to 1. Also, the message is expected to be sent every 50 ms approximatively. If this
      | condition is not met 5 times consecutively the 'TX Warn' output is set to 1.
  TX status : Inport
  TX delta time : Inport  Port=2
  Delta time limit : Constant  Value=0.055
  Delta time limit exceeded : RelationalOperator  RndMeth=Nearest  InputSameDT=on
  Mem{1..4} (4 alike) : Memory
  OR : Logic  Operator=OR
  Prev. msg. not sent : RelationalOperator  Operator=~=  RndMeth=Nearest  InputSameDT=on
  Prev. msg. sent value : Constant
  Warn : Logic  Inputs=5
  TX Warn : Outport
  wires:
  TX delta time/1 -> Delta time limit exceeded/1
  Delta time limit/1 -> Delta time limit exceeded/2
  Prev. msg. sent value/1 -> Prev. msg. not sent/2
  TX status/1 -> Prev. msg. not sent/1
  Prev. msg. not sent/1 -> OR/1
  Delta time limit exceeded/1 -> OR/2
  OR/1 -> Mem1/1, Warn/1
  Mem1/1 -> Mem2/1, Warn/2
  Mem2/1 -> Mem3/1, Warn/3
  Mem3/1 -> Mem4/1, Warn/4
  Mem4/1 -> Warn/5
  Warn/1 -> TX Warn/1

== system Framework/Subsystem2/Transmit OK Detection7 ==
  note: This subsystem surveys if the sending of the TX message is successful and if it meets the
      | requirements concerning the regularity of the sending.
      |
      | If for 5 consecutive execution steps the message could not be successfully sent the 'TX Warn'
      | output is set to 1. Also, the message is expected to be sent every 50 ms approximatively. If this
      | condition is not met 5 times consecutively the 'TX Warn' output is set to 1.
  TX status : Inport
  TX delta time : Inport  Port=2
  Delta time limit : Constant  Value=0.055
  Delta time limit exceeded : RelationalOperator  RndMeth=Nearest  InputSameDT=on
  Mem{1..4} (4 alike) : Memory
  OR : Logic  Operator=OR
  Prev. msg. not sent : RelationalOperator  Operator=~=  RndMeth=Nearest  InputSameDT=on
  Prev. msg. sent value : Constant
  Warn : Logic  Inputs=5
  TX Warn : Outport
  wires:
  TX delta time/1 -> Delta time limit exceeded/1
  Delta time limit/1 -> Delta time limit exceeded/2
  Prev. msg. sent value/1 -> Prev. msg. not sent/2
  TX status/1 -> Prev. msg. not sent/1
  Prev. msg. not sent/1 -> OR/1
  Delta time limit exceeded/1 -> OR/2
  OR/1 -> Mem1/1, Warn/1
  Mem1/1 -> Mem2/1, Warn/2
  Mem2/1 -> Mem3/1, Warn/3
  Mem3/1 -> Mem4/1, Warn/4
  Mem4/1 -> Warn/5
  Warn/1 -> TX Warn/1

== system Framework/Subsystem2/Transmit OK Detection9 ==
  note: This subsystem surveys if the sending of the TX message is successful and if it meets the
      | requirements concerning the regularity of the sending.
      |
      | If for 5 consecutive execution steps the message could not be successfully sent the 'TX Warn'
      | output is set to 1. Also, the message is expected to be sent every 50 ms approximatively. If this
      | condition is not met 5 times consecutively the 'TX Warn' output is set to 1.
  TX status : Inport
  TX delta time : Inport  Port=2
  Delta time limit : Constant  Value=0.055
  Delta time limit exceeded : RelationalOperator  RndMeth=Nearest  InputSameDT=on
  Mem{1..4} (4 alike) : Memory
  OR : Logic  Operator=OR
  Prev. msg. not sent : RelationalOperator  Operator=~=  RndMeth=Nearest  InputSameDT=on
  Prev. msg. sent value : Constant
  Warn : Logic  Inputs=5
  TX Warn : Outport
  wires:
  TX delta time/1 -> Delta time limit exceeded/1
  Delta time limit/1 -> Delta time limit exceeded/2
  Prev. msg. sent value/1 -> Prev. msg. not sent/2
  TX status/1 -> Prev. msg. not sent/1
  Prev. msg. not sent/1 -> OR/1
  Delta time limit exceeded/1 -> OR/2
  OR/1 -> Mem1/1, Warn/1
  Mem1/1 -> Mem2/1, Warn/2
  Mem2/1 -> Mem3/1, Warn/3
  Mem3/1 -> Mem4/1, Warn/4
  Mem4/1 -> Warn/5
  Warn/1 -> TX Warn/1

== system Framework/Subsystem3/Transmit OK Detection10 ==
  note: This subsystem surveys if the sending of the TX message is successful and if it meets the
      | requirements concerning the regularity of the sending.
      |
      | If for 5 consecutive execution steps the message could not be successfully sent the 'TX Warn'
      | output is set to 1. Also, the message is expected to be sent every 50 ms approximatively. If this
      | condition is not met 5 times consecutively the 'TX Warn' output is set to 1.
  TX status : Inport
  TX delta time : Inport  Port=2
  Delta time limit : Constant  Value=0.055
  Delta time limit exceeded : RelationalOperator  RndMeth=Nearest  InputSameDT=on
  Mem{1..4} (4 alike) : Memory
  OR : Logic  Operator=OR
  Prev. msg. not sent : RelationalOperator  Operator=~=  RndMeth=Nearest  InputSameDT=on
  Prev. msg. sent value : Constant
  Warn : Logic  Inputs=5
  TX Warn : Outport
  wires:
  TX delta time/1 -> Delta time limit exceeded/1
  Delta time limit/1 -> Delta time limit exceeded/2
  Prev. msg. sent value/1 -> Prev. msg. not sent/2
  TX status/1 -> Prev. msg. not sent/1
  Prev. msg. not sent/1 -> OR/1
  Delta time limit exceeded/1 -> OR/2
  OR/1 -> Mem1/1, Warn/1
  Mem1/1 -> Mem2/1, Warn/2
  Mem2/1 -> Mem3/1, Warn/3
  Mem3/1 -> Mem4/1, Warn/4
  Mem4/1 -> Warn/5
  Warn/1 -> TX Warn/1

== system Framework/Subsystem3/Transmit OK Detection8 ==
  note: This subsystem surveys if the sending of the TX message is successful and if it meets the
      | requirements concerning the regularity of the sending.
      |
      | If for 5 consecutive execution steps the message could not be successfully sent the 'TX Warn'
      | output is set to 1. Also, the message is expected to be sent every 50 ms approximatively. If this
      | condition is not met 5 times consecutively the 'TX Warn' output is set to 1.
  TX status : Inport
  TX delta time : Inport  Port=2
  Delta time limit : Constant  Value=0.055
  Delta time limit exceeded : RelationalOperator  RndMeth=Nearest  InputSameDT=on
  Mem{1..4} (4 alike) : Memory
  OR : Logic  Operator=OR
  Prev. msg. not sent : RelationalOperator  Operator=~=  RndMeth=Nearest  InputSameDT=on
  Prev. msg. sent value : Constant
  Warn : Logic  Inputs=5
  TX Warn : Outport
  wires:
  TX delta time/1 -> Delta time limit exceeded/1
  Delta time limit/1 -> Delta time limit exceeded/2
  Prev. msg. sent value/1 -> Prev. msg. not sent/2
  TX status/1 -> Prev. msg. not sent/1
  Prev. msg. not sent/1 -> OR/1
  Delta time limit exceeded/1 -> OR/2
  OR/1 -> Mem1/1, Warn/1
  Mem1/1 -> Mem2/1, Warn/2
  Mem2/1 -> Mem3/1, Warn/3
  Mem3/1 -> Mem4/1, Warn/4
  Mem4/1 -> Warn/5
  Warn/1 -> TX Warn/1

== system Framework/duty cycle FL/Transmit OK Detection ==
  note: This subsystem surveys if the sending of the TX message is successful and if it meets the
      | requirements concerning the regularity of the sending.
      |
      | If for 5 consecutive execution steps the message could not be successfully sent the 'TX Warn'
      | output is set to 1. Also, the message is expected to be sent every 50 ms approximatively. If this
      | condition is not met 5 times consecutively the 'TX Warn' output is set to 1.
  TX status : Inport
  TX delta time : Inport  Port=2
  Delta time limit : Constant  Value=0.055
  Delta time limit exceeded : RelationalOperator  RndMeth=Nearest  InputSameDT=on
  Mem{1..4} (4 alike) : Memory
  OR : Logic  Operator=OR
  Prev. msg. not sent : RelationalOperator  Operator=~=  RndMeth=Nearest  InputSameDT=on
  Prev. msg. sent value : Constant
  Warn : Logic  Inputs=5
  TX Warn : Outport
  wires:
  TX delta time/1 -> Delta time limit exceeded/1
  Delta time limit/1 -> Delta time limit exceeded/2
  Prev. msg. sent value/1 -> Prev. msg. not sent/2
  TX status/1 -> Prev. msg. not sent/1
  Prev. msg. not sent/1 -> OR/1
  Delta time limit exceeded/1 -> OR/2
  OR/1 -> Mem1/1, Warn/1
  Mem1/1 -> Mem2/1, Warn/2
  Mem2/1 -> Mem3/1, Warn/3
  Mem3/1 -> Mem4/1, Warn/4
  Mem4/1 -> Warn/5
  Warn/1 -> TX Warn/1

== system Framework/duty cycle FR/Transmit OK Detection ==
  note: This subsystem surveys if the sending of the TX message is successful and if it meets the
      | requirements concerning the regularity of the sending.
      |
      | If for 5 consecutive execution steps the message could not be successfully sent the 'TX Warn'
      | output is set to 1. Also, the message is expected to be sent every 50 ms approximatively. If this
      | condition is not met 5 times consecutively the 'TX Warn' output is set to 1.
  TX status : Inport
  TX delta time : Inport  Port=2
  Delta time limit : Constant  Value=0.055
  Delta time limit exceeded : RelationalOperator  RndMeth=Nearest  InputSameDT=on
  Mem{1..4} (4 alike) : Memory
  OR : Logic  Operator=OR
  Prev. msg. not sent : RelationalOperator  Operator=~=  RndMeth=Nearest  InputSameDT=on
  Prev. msg. sent value : Constant
  Warn : Logic  Inputs=5
  TX Warn : Outport
  wires:
  TX delta time/1 -> Delta time limit exceeded/1
  Delta time limit/1 -> Delta time limit exceeded/2
  Prev. msg. sent value/1 -> Prev. msg. not sent/2
  TX status/1 -> Prev. msg. not sent/1
  Prev. msg. not sent/1 -> OR/1
  Delta time limit exceeded/1 -> OR/2
  OR/1 -> Mem1/1, Warn/1
  Mem1/1 -> Mem2/1, Warn/2
  Mem2/1 -> Mem3/1, Warn/3
  Mem3/1 -> Mem4/1, Warn/4
  Mem4/1 -> Warn/5
  Warn/1 -> TX Warn/1

== system Framework/duty cycle RL/Transmit OK Detection ==
  note: This subsystem surveys if the sending of the TX message is successful and if it meets the
      | requirements concerning the regularity of the sending.
      |
      | If for 5 consecutive execution steps the message could not be successfully sent the 'TX Warn'
      | output is set to 1. Also, the message is expected to be sent every 50 ms approximatively. If this
      | condition is not met 5 times consecutively the 'TX Warn' output is set to 1.
  TX status : Inport
  TX delta time : Inport  Port=2
  Delta time limit : Constant  Value=0.055
  Delta time limit exceeded : RelationalOperator  RndMeth=Nearest  InputSameDT=on
  Mem{1..4} (4 alike) : Memory
  OR : Logic  Operator=OR
  Prev. msg. not sent : RelationalOperator  Operator=~=  RndMeth=Nearest  InputSameDT=on
  Prev. msg. sent value : Constant
  Warn : Logic  Inputs=5
  TX Warn : Outport
  wires:
  TX delta time/1 -> Delta time limit exceeded/1
  Delta time limit/1 -> Delta time limit exceeded/2
  Prev. msg. sent value/1 -> Prev. msg. not sent/2
  TX status/1 -> Prev. msg. not sent/1
  Prev. msg. not sent/1 -> OR/1
  Delta time limit exceeded/1 -> OR/2
  OR/1 -> Mem1/1, Warn/1
  Mem1/1 -> Mem2/1, Warn/2
  Mem2/1 -> Mem3/1, Warn/3
  Mem3/1 -> Mem4/1, Warn/4
  Mem4/1 -> Warn/5
  Warn/1 -> TX Warn/1
